simulink model "Q4_LQG"  (R2019b)
settings: Solver=FixedStepAuto  StartTime=0.0  StopTime=6  FixedStep=0.01  RelTol=1e-3
undefined symbols (not defined in the file or in its folder): Continuous, Time
libraries: ctrlSharedLib x1
settings Model: Creator=allen  LastModifiedBy=allen

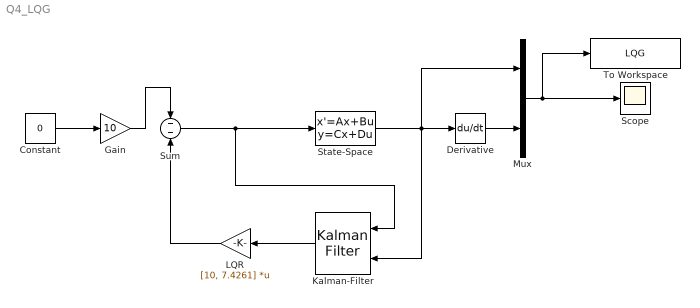
== system Q4_LQG ==
  Constant : Constant  Value=0
  Derivative : Derivative
  Gain : Gain  Gain=10
  Kalman-Filter : ctrlSharedLib/Kalman Filter  TimeDomain=Continuous-Time  UseCurrentEstimator=on  ModelSource=Individual A, B, C, D matrices  ModelSourceVariable=ss(0.95,1,1,0,1)  A=[0 1;0 -1]  B=[0;1]  C=[1 0]  D=0  NumberOfStates=1  NumberOfInputs=1  NumberOfOutputs=1  InitialEstimateSource=Dialog  X0=[0;0]  P0=10  UseK=off  UseGH=off  NumberOfProcessNoiseInputs=1  G=1  TimeInvariantG=on  H=0  TimeInvariantH=on  Q=[1 0;0 0]  TimeInvariantQ=on  R=0.2  TimeInvariantR=on  N=0  TimeInvariantN=on  AddInputPort=on  AddEnablePort=off  OutputEstimatedY=off  OutputP=off  Ts=-1
      settings: SourceProductBaseCode=CT
  LQR : Gain  Gain=[10, 7.4261]  Multiplication=Matrix(K*u)
  Mux : Mux  Inputs=2
  Scope : Scope
  State-Space : StateSpace  A=[0 1;0 -1]  B=[0;1]  C=[1 0]  D=0  InitialCondition=[1;0.5]
  Sum : Sum  Inputs=--
  To Workspace : ToWorkspace  VariableName=LQG  SampleTime=-1
  wires:
  State-Space/1 -> Kalman-Filter/2, Derivative/1, Mux/1
  Kalman-Filter/1 -> LQR/1
  LQR/1 -> Sum/2
  Constant/1 -> Gain/1
  Gain/1 -> Sum/1
  Sum/1 -> Kalman-Filter/1, State-Space/1
  Derivative/1 -> Mux/2
  Mux/1 -> To Workspace/1, Scope/1
